simulink model "Lab_6"  (R2022b)
settings: Solver=VariableStepAuto  StartTime=0.0  StopTime=300.0  RelTol=1e-3
undefined symbols (not defined in the file): h, SP, T, tau
settings Model: Creator=janro  LastModifiedBy=janro

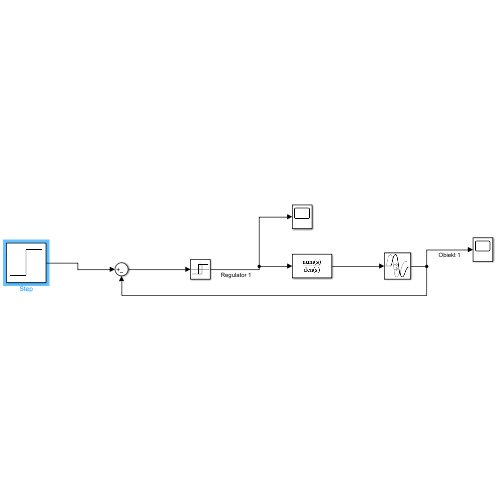
[thumbnail: Simulink's stored preview of the top-level diagram]
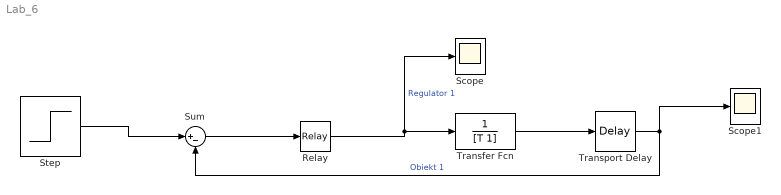
== system Lab_6 ==
  Relay : Relay  OnSwitchValue=h  OffSwitchValue=-h
  Scope : Scope
  Scope1 : Scope
  Step : Step  Time=0  After=SP  SampleTime=0
  Sum : Sum  Inputs=|+-
  Transfer Fcn : TransferFcn  Numerator=[0 1]  Denominator=[T 1]
  Transport Delay : TransportDelay  DelayTime=tau  PadeOrder=10
  wires:
  Step/1 -> Sum/1
  Sum/1 -> Relay/1
  Relay/1 -> Scope/1, Transfer Fcn/1  "Regulator 1"
  Transfer Fcn/1 -> Transport Delay/1
  Transport Delay/1 -> Sum/2, Scope1/1  "Obiekt 1"
